simulink model "ExperimentalCarrier_lateral"  (R2015b)
settings: Solver=ode45  StartTime=0.0  StopTime=60  FixedStep=0.001  RelTol=1e-4
model workspace (MAT data in the model file):
  CX = [-0.0337179757175 -0.0333639962938 -0.0333029382182 -0.0332484475689 -0.0332754358974 -0.0333222022118 -0.0336346734879]
  CX_P = [-0.00180360991901 0.00664184177361 -2.42842311075e-05 -2.06955249234e-05 0.000107673639449 -0.00557660802406 0.00168313316358]
  CX_Q = [-0.276174674886 -0.276045033417 -0.276727133168 -0.276868141641 -0.276462581291 -0.275997191298 -0.275111306167]
  CX_R = [0.00609178533876 0.0032136083659 0.00288050935178 0.00139231210283 -0.000188148946793 -0.000699030607472 -0.00363844024964]
  CX_d = reshape([-0.0225280716674 -0.0223891508479 -0.0223681780505 -0.0223432519069 -0.0222296413505 -0.0221761942058 -0.0220710295662 0.00600012359207 0.00559383606852 0.00521927991354 0.00484253129263 0.00441803454099 0.00422262712747 0.00373799149772], [1 7 2])
  CX_d_elevator = [-0.0225280716674 -0.0223891508479 -0.0223681780505 -0.0223432519069 -0.0222296413505 -0.0221761942058 -0.0220710295662]
  CX_d_rudder = [0.00600012359207 0.00559383606852 0.00521927991354 0.00484253129263 0.00441803454099 0.00422262712747 0.00373799149772]
  CY = [0.0172529817358 0.011982932276 0.00606303689375 0.00025383868563 -0.00547298868785 -0.0111687863685 -0.0165472100647]
  CY_P = [0.374118009617 0.39290598718 0.381365334981 0.374685279781 0.377426336703 0.381898667412 0.372668227194]
  CY_Q = [0.150901852738 0.143298654224 0.128022476676 0.113476069408 0.0995119426864 0.0857134029 0.0760386872967]
  CY_R = [-0.333129286686 -0.332948508644 -0.33123397315 -0.329896924353 -0.32907206565 -0.328546079974 -0.32737851652]
  CY_d = reshape([0.0196606436595 0.0184850450981 0.0169055682098 0.0153372661358 0.0138073476115 0.0123331166649 0.0110240247349 -0.141169320798 -0.140142140967 -0.139060957332 -0.137968433842 -0.136853005187 -0.135813824899 -0.134831648888], [1 7 2])
  CY_d_elevator = [0.0196606436595 0.0184850450981 0.0169055682098 0.0153372661358 0.0138073476115 0.0123331166649 0.0110240247349]
  CY_d_rudder = [-0.141169320798 -0.140142140967 -0.139060957332 -0.137968433842 -0.136853005187 -0.135813824899 -0.134831648888]
  CZ = [0.534699164694 0.533477327658 0.533357818874 0.533162719235 0.532815330236 0.53255803197 0.533058072044]
  CZ_P = [-0.00329431835884 -0.0312298742688 -0.0131618738693 0.00139526572222 0.0131110439838 0.0227220539184 0.00563920214525]
  CZ_Q = [7.41132042869 7.41242879879 7.42202221037 7.42972491576 7.43439811242 7.43851081289 7.44797822831]
  CZ_R = [-0.0560788369874 -0.0469826195755 -0.040186761785 -0.0328451122892 -0.0248853142685 -0.0162626721689 -0.00562389662543]
  CZ_d = reshape([0.556183511159 0.556588453756 0.557396308141 0.558052886154 0.558502738673 0.558892777679 0.559544685718 -0.108954693177 -0.107634840368 -0.106474972402 -0.105298511014 -0.104084914231 -0.102894555312 -0.101853973024], [1 7 2])
  CZ_d_elevator = [0.556183511159 0.556588453756 0.557396308141 0.558052886154 0.558502738673 0.558892777679 0.559544685718]
  CZ_d_rudder = [-0.108954693177 -0.107634840368 -0.106474972402 -0.105298511014 -0.104084914231 -0.102894555312 -0.101853973024]
  Cl = [-0.00700764664959 -0.00472973282884 -0.00237582843662 -2.25913583358e-05 0.00233475877084 0.00469949778092 0.00703390515758]
  Cl_P = [-0.44204167247 -0.444124298051 -0.443158723294 -0.442636624151 -0.44302101642 -0.443480587262 -0.44220785431]
  Cl_Q = [-0.00761433176316 -0.00871202586947 -0.00915701177502 -0.00960939426583 -0.0100395709176 -0.0104261696426 -0.0111166239143]
  Cl_R = [0.0702655648896 0.0705743616107 0.0707504085215 0.0709698715526 0.0712606870971 0.0715881820975 0.0718747336385]
  Cl_d = reshape([-0.00146489638275 -0.00143738931585 -0.00137422415916 -0.00130841024919 -0.00123816152715 -0.00116289316043 -0.00109913093002 0.0123681436285 0.0122704324373 0.0121659224143 0.0120592912182 0.0119488136709 0.011839351441 0.0117379077047], [1 7 2])
  Cl_d_elevator = [-0.00146489638275 -0.00143738931585 -0.00137422415916 -0.00130841024919 -0.00123816152715 -0.00116289316043 -0.00109913093002]
  Cl_d_rudder = [0.0123681436285 0.0122704324373 0.0121659224143 0.0120592912182 0.0119488136709 0.011839351441 0.0117379077047]
  Cm = [-0.00401015961928 -0.000975274975777 -0.00046553481727 4.4136183697e-05 0.000715039140208 0.0010246745677 -0.000455960949925]
  Cm_P = [0.0363979880935 0.0870326194808 0.0380519486412 -0.00305191920923 -0.0379708477237 -0.0686773821057 -0.0415582211907]
  Cm_Q = [-9.31033666478 -9.31035016738 -9.32990293705 -9.34666189261 -9.35805453149 -9.36965047911 -9.39387328022]
  Cm_R = [0.121087302826 0.101546010828 0.0872107966775 0.0715178778578 0.0544215297596 0.0359658689904 0.0128153299816]
  Cm_d = reshape([-1.26563318748 -1.26652764985 -1.26830421062 -1.26977092408 -1.27078647089 -1.27170767282 -1.27318033181 0.238605889367 0.235644018015 0.23304116627 0.230407854048 0.227691183297 0.225077263964 0.222740695151], [1 7 2])
  Cm_d_elevator = [-1.26563318748 -1.26652764985 -1.26830421062 -1.26977092408 -1.27078647089 -1.27170767282 -1.27318033181]
  Cm_d_rudder = [0.238605889367 0.235644018015 0.23304116627 0.230407854048 0.227691183297 0.225077263964 0.222740695151]
  Cn = [0.00334100631412 0.00240143469011 0.00123926351105 0.000107729711747 -0.000988454643432 -0.00205913402605 -0.00303968727266]
  Cn_P = [-0.00770316035359 -0.00146703051444 -0.00502111646166 -0.00766050784277 -0.00674014018918 -0.00597496765186 -0.00838382166573]
  Cn_Q = [0.0596503718601 0.0577019150227 0.0528770013595 0.0482559644739 0.0438602730584 0.0395011779308 0.0366194045402]
  Cn_R = [-0.115202541198 -0.114925014185 -0.114354791039 -0.113787196313 -0.113397645546 -0.112981789027 -0.112619149701]
  Cn_d = reshape([0.00791652254186 0.00755393552521 0.00703679063877 0.00652453082009 0.00602668569172 0.00554077748029 0.00511800575953 -0.0599631923684 -0.0595911197493 -0.0591978291139 -0.0588022387871 -0.0584016103277 -0.0580069864684 -0.0576675613767], [1 7 2])
  Cn_d_elevator = [0.00791652254186 0.00755393552521 0.00703679063877 0.00652453082009 0.00602668569172 0.00554077748029 0.00511800575953]
  Cn_d_rudder = [-0.0599631923684 -0.0595911197493 -0.0591978291139 -0.0588022387871 -0.0584016103277 -0.0580069864684 -0.0576675613767]
  InertiaTensor = [1  0  0; 0  1  0; 0  0  1]
  aircraft_geometry_name = 'ExperimentalCarrier'
  alpha = 0.0912564214814
  beta = [-0.0349065850399; -0.0232710566933; -0.0116355283466; 0; 0.0116355283466; 0.0232710566933; 0.0349065850399]
  centerOfGravity = -0.092
  estimatedVelocity = 14
  mass = 1.56
  mean_chord = 0.25
  p_ini = 0
  phi_ini = 0
  psi_ini = 0
  r_ini = 0
  spanwidth = 1.5
  theta_ini = 0.0624021030233
  u_ini = 11.5418432655
  v_ini = 0
  w_ini = 1.05620086286
undefined symbols (not defined in the file): Earth, eul_0, m, pm_0, s, Vm_0, WGS84
libraries: aerolibconvert2 x6, aerolib6dofsys x2, aerolibtransform2 x2, aerolibasang x2, aerolibfltsims x2, aerolibutil x1, aerolibadyn x1, aerolibanimutils x1, aerolibatmos2 x1, aerolibgravity2 x1
settings Model: Creator=jruesch  LastModifiedBy=jruesch
settings DataIOCC: SaveFormat=Array
settings OptimizationCC: BlockReduction=off
settings HardwareCC: ProdBitPerPointer=32  ProdLargestAtomicFloat=None  ProdIntDivRoundTo=Undefined  ProdEndianess=Unspecified  ProdWordSize=32  ProdHWDeviceType=32-bit Generic
settings GRTTargetCC: GeneratePreprocessorConditionals=Disable all
settings ConfigComp: CovModelRefEnable=Off

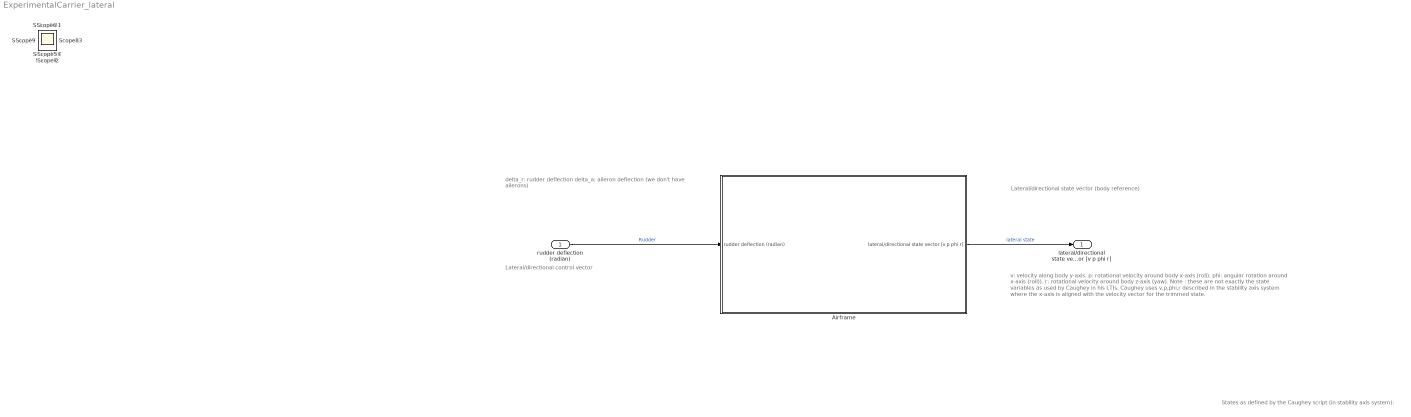
== system ExperimentalCarrier_lateral ==
  note: delta_r: rudder deflection
      | delta_a: aileron deflection (we don't have ailerons)
  note: Lateral/directional control vector
  note: v: velocity along body y-axis.
      | p: rotational velocity around body x-axis (roll).
      | phi: angular rotation around x-axis (roll)).
      | r: rotational velocity around body z-axis (yaw).
      |
      | Note : these are not exactly the state variables as used by Caughey in his LTIs.
      | Caughey uses v,p,phi,r described in the stability axis system where the x-axis is aligned
      | with the velocity vector for the trimmed state.
  note: Lateral/directional state vector (body reference)
  note: States as defined by the Caughey script (in stability axis system):
  rudder deflection (radian) : Inport
  Airframe : Subsystem
      mask Display: image(imread('../../figures/Airframe01.png'))
  lateral/directional state vector [v p phi r] : Outport
  Scope{,1..44} (45 alike) : Scope
  wires:
  rudder deflection (radian)/1 -> Airframe/1(rudder deflection (radian))  "Rudder"
  Airframe/1(lateral/directional state vector [v p phi r]) -> lateral/directional state vector [v p phi r]/1  "lateral state"

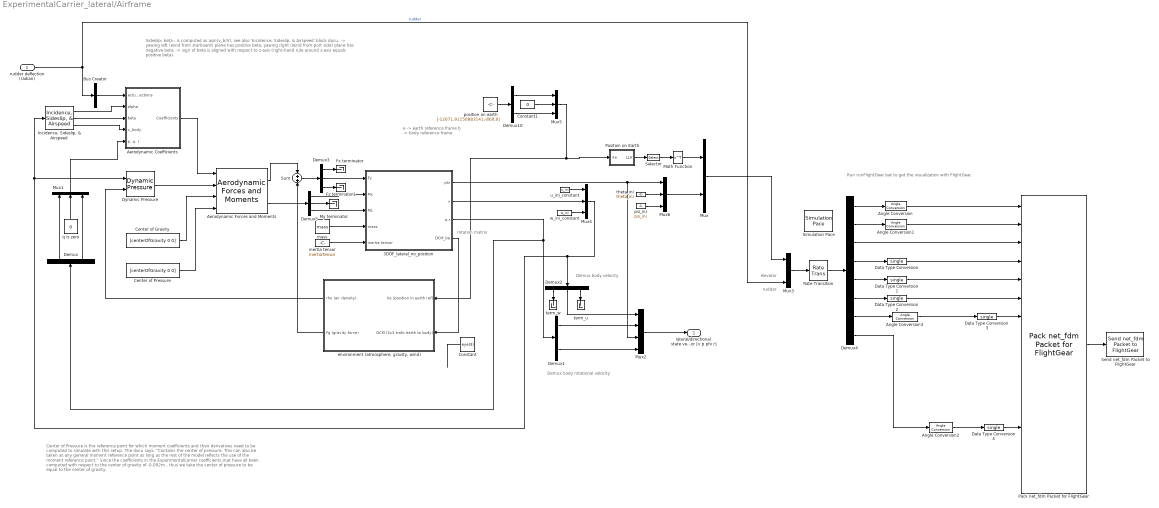
== system ExperimentalCarrier_lateral/Airframe ==
  note: rotation matrix
  note: rudder
  note: elevator
  note: Sideslip:
      | beta : is computed as asin(v_b/V), see also 'Incidence, Sideslip, & Airspeed' block docu.
      | -> yawing left (wind from starboard) plane has positive beta, yawing right (wind from port side) plane has negative beta.
      | -> sign of beta is aligned with respect to z-axis (right-hand rule around z-axis equals positive beta).
  note: Demux body velocity
  note: Run runFlightGear.bat to get the visualization with FlightGear.
  note: e -> earth reference frame
      | b -> body reference frame
  note: Center of Pressure is the reference point for which moment coefficients and their derivatives need to be computed to simulate with this setup.
      | The docu says: "Contains the center of pressure. This can also be taken as any general moment reference point as long as the rest of the model
      | reflects the use of the moment reference point." Since the coefficients in the ExperimentalCarrier coefficients.mat have all been computed with respect to
      | the center of gravity of -0.092m , thus we take the center of pressure to be equal to the center of gravity.
  note: Demux body rotational velocity
  rudder deflection (radian) : Inport
  3DOF_lateral_no_position : Subsystem
  "Aerodynamic Forces and Moments " : aerolibadyn/Aerodynamic Forces and Moments   inputAxes=Body  outputForceAxes=Body  outputMomentAxes=Body  S=spanwidth*mean_chord  b=spanwidth  cbar=mean_chord
  Aerodynamic Coefficients : Subsystem
  Angle Conversion : aerolibconvert2/Angle Conversion  IU=deg  OU=rad
  Angle Conversion1 : aerolibconvert2/Angle Conversion  IU=deg  OU=rad
  Angle Conversion2 : aerolibconvert2/Angle Conversion  IU=rad  OU=deg
  Angle Conversion3 : aerolibconvert2/Angle Conversion  IU=rad  OU=deg
  Bus Creator : BusCreator  Inputs=1
  Center of Gravity : Constant  Value=[centerOfGravity 0 0]
  Center of Pressure : Constant  Value=[centerOfGravity 0 0]
  Constant : Constant  Value=eye(3)
  Constant1 : Constant  Value=0
  Data Type Conversion{,1..4} (5 alike) : DataTypeConversion  OutDataTypeStr=single
  Demux : Demux  Outputs=2
  Demux1 : Demux  Outputs=2
  Demux10 : Demux  Outputs=2
  Demux2 : Demux  Outputs=3
  Demux3 : Demux  Outputs=3
  Demux4 : Demux  Outputs=8
  Demux5 : Demux  Outputs=3
  Dynamic Pressure : aerolibasang/Dynamic Pressure
  Fx terminator : Terminator
  Fz terminator1 : Terminator
  "Incidence, Sideslip, & Airspeed" : aerolibasang/Incidence, Sideslip, & Airspeed
  Math Function : Math  Operator=transpose  SaturateOnIntegerOverflow=on
  Mux : Mux  Inputs=2
  Mux{1,3..6} (5 alike) : Mux  Inputs=3
  Mux2 : Mux
  My terminator : Terminator
  Pack net_fdm Packet for FlightGear : aerolibfltsims/Pack net_fdm Packet for FlightGear  FlightGearVersion=v3.4  ShowPositionAttitudeInputs=on  ShowVelocityAccelerationInputs=off  ShowControlSurfacePositionInputs=on  ShowEngineFuelInputs=off  ShowLandingGearInputs=off  ShowEnvironmentInputs=off  SampleTime=1/30
  Position on Earth : Subsystem  Priority=1  TreatAsAtomicUnit=on
  Rate Transition : RateTransition  Integrity=off  OutPortSampleTime=1/30
  Selector : Selector  InputPortWidth=3  IndexOptions=Index vector (dialog)  Indices=[2 1 3]  OutputSizes=1
  Send net_fdm Packet to FlightGear : aerolibfltsims/Send net_fdm Packet to FlightGear  DestinationIpAddress=127.0.0.1  DestinationPort=5502  LocalIpPort=-1  varLen=off  SampleTime=1/30
  Simulation Pace : aerolibanimutils/Simulation Pace  SimulationPace=1  SleepMode=MATLAB Thread  OutputPaceError=off  SampleTime=1/30
      settings: AttributesFormatString=%<SimulationPace> sec/sec
  Sum : Sum
  "environment (atmosphere, gravity, wind)" : Subsystem
  inertia tensor : Constant  Value=InertiaTensor
  mass : Constant  Value=mass
  position on earth : Constant  Value=[-12071.91150883141;-800.0]
  psi_ini : Constant  Value=psi_ini
  q is zero : Constant  Value=0
  term_u : Terminator
  term_w : Terminator
  theta_ini : Constant  Value=theta_ini
  u_ini_constant : Constant  Value=u_ini
  w_ini_constant : Constant  Value=w_ini
  lateral/directional state vector [v p phi r] : Outport
  wires:
  "Aerodynamic Forces and Moments "/1 -> Sum/1
  "Aerodynamic Forces and Moments "/2 -> Demux5/1
  Center of Gravity/1 -> "Aerodynamic Forces and Moments "/3
  Center of Pressure/1 -> "Aerodynamic Forces and Moments "/4
  Dynamic Pressure/1 -> "Aerodynamic Forces and Moments "/2
  Position on Earth/1(LLA) -> Selector/1
  3DOF_lateral_no_position/4(DCM_be) -> "environment (atmosphere, gravity, wind)"/2(DCM (3x3 trafo earth to body))
  3DOF_lateral_no_position/1(phi) -> Mux6/1, Mux2/3
  Mux4/1 -> Demux2/1, "Incidence, Sideslip, & Airspeed"/1, Dynamic Pressure/1
  3DOF_lateral_no_position/3(p,r) -> Demux/1, Demux1/1
  Math Function/1 -> Mux/1
  Mux/1 -> Mux3/1
  Selector/1 -> Math Function/1
  "environment (atmosphere, gravity, wind)"/1(rho (air density)) -> Dynamic Pressure/2
  "environment (atmosphere, gravity, wind)"/2(Fg (gravity force)) -> Sum/2
  "Incidence, Sideslip, & Airspeed"/2 -> Aerodynamic Coefficients/3(beta)
  "Incidence, Sideslip, & Airspeed"/3 -> Aerodynamic Coefficients/4(v_body)
  Aerodynamic Coefficients/1(Coefficients) -> "Aerodynamic Forces and Moments "/1
  Bus Creator/1 -> Aerodynamic Coefficients/1(actuator deflections)
  rudder deflection (radian)/1 -> Bus Creator/1, Mux3/3  "rudder"
  Sum/1 -> Demux3/1
  Demux1/1 -> Mux2/2
  Mux2/1 -> lateral/directional state vector [v p phi r]/1
  Pack net_fdm Packet for FlightGear/1 -> Send net_fdm Packet to FlightGear/1
  Demux4/1 -> Angle Conversion/1
  Demux4/2 -> Angle Conversion1/1
  Demux4/3 -> Pack net_fdm Packet for FlightGear/3
  Demux4/4 -> Data Type Conversion/1
  Demux4/5 -> Data Type Conversion1/1
  Demux4/6 -> Data Type Conversion2/1
  Rate Transition/1 -> Demux4/1
  Angle Conversion/1 -> Pack net_fdm Packet for FlightGear/1
  Angle Conversion1/1 -> Pack net_fdm Packet for FlightGear/2
  Data Type Conversion/1 -> Pack net_fdm Packet for FlightGear/4
  Data Type Conversion1/1 -> Pack net_fdm Packet for FlightGear/5
  Data Type Conversion2/1 -> Pack net_fdm Packet for FlightGear/6
  Mux3/1 -> Rate Transition/1
  Demux4/7 -> Angle Conversion3/1
  Demux4/8 -> Angle Conversion2/1
  Data Type Conversion3/1 -> Pack net_fdm Packet for FlightGear/7
  Data Type Conversion4/1 -> Pack net_fdm Packet for FlightGear/13
  Angle Conversion2/1 -> Data Type Conversion4/1
  Angle Conversion3/1 -> Data Type Conversion3/1
  inertia tensor/1 -> 3DOF_lateral_no_position/5(inertia tensor)
  mass/1 -> 3DOF_lateral_no_position/4("mass ")
  Constant1/1 -> Mux5/2
  position on earth/1 -> Demux10/1
  Demux10/2 -> Mux5/3
  Demux10/1 -> Mux5/1
  Mux5/1 -> Position on Earth/1(Xe), "environment (atmosphere, gravity, wind)"/1(Xe (position in earth ref))
  Demux3/2 -> 3DOF_lateral_no_position/1(Fy)
  Demux5/1 -> 3DOF_lateral_no_position/2(Mx)
  Demux5/3 -> 3DOF_lateral_no_position/3(Mz)
  Demux5/2 -> My terminator/1
  Demux3/1 -> Fx terminator/1
  Demux3/3 -> Fz terminator1/1
  Demux1/2 -> Mux2/4
  Demux/1 -> Mux1/1
  Demux/2 -> Mux1/3
  Mux1/1 -> Aerodynamic Coefficients/5("p, q, r")
  q is zero/1 -> Mux1/2
  w_ini_constant/1 -> Mux4/3
  u_ini_constant/1 -> Mux4/1
  3DOF_lateral_no_position/2(v) -> Mux4/2
  theta_ini/1 -> Mux6/2
  psi_ini/1 -> Mux6/3
  Mux6/1 -> Mux/2
  Demux2/2 -> Mux2/1
  Demux2/1 -> term_w/1
  Demux2/3 -> term_u/1
  Constant/1 -> ?
  "Incidence, Sideslip, & Airspeed"/1 -> Aerodynamic Coefficients/2(alpha)

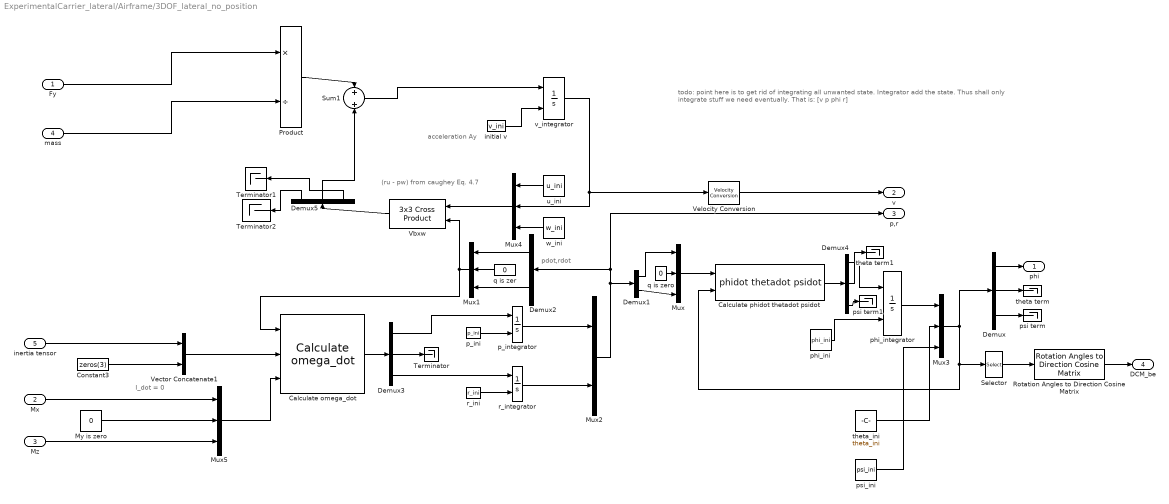
== system ExperimentalCarrier_lateral/Airframe/3DOF_lateral_no_position ==
  note: (ru - pw)
      | from caughey Eq. 4.7
  note: I_dot = 0
  note: todo: point here is to get rid of integrating all unwanted state.
      | Integrator add the state. Thus shall only integrate stuff we need
      | eventually. That is: [v p phi r]
  note: pdot,rdot
  note: acceleration Ay
  Fy : Inport
  Mx : Inport  Port=2  PortDimensions=1
  Mz : Inport  Port=3  PortDimensions=1
  "mass " : Inport  Port=4
  inertia tensor : Inport  Port=5
  Calculate omega_dot : aerolib6dofsys/Calculate omega_dot  SystemSampleTime=-1
  Calculate phidot thetadot psidot : aerolib6dofsys/DCM & Euler Angles (Euler)/phidot thetadot psidot
  Constant3 : Constant  Value=zeros(3)
  Demux{,3..5} (4 alike) : Demux  Outputs=3
  Demux1 : Demux  Outputs=2
  Demux2 : Demux  Outputs=2
  Mux{,1,3..5} (5 alike) : Mux  Inputs=3
  Mux2 : Mux  Inputs=2
  My is zero : Constant  Value=0
  Product : Product  Inputs=*/  SaturateOnIntegerOverflow=on  OutDataTypeStr=Inherit: Same as first input
  Rotation Angles to Direction Cosine Matrix : aerolibtransform2/Rotation Angles to Direction Cosine Matrix  rotationOrder=ZYX
  Selector : Selector  InputPortWidth=3  IndexOptions=Index vector (dialog)  Indices=[3 2 1]  OutputSizes=1
  Sum1 : Sum  SaturateOnIntegerOverflow=on
  Terminator : Terminator
  Terminator1 : Terminator
  Terminator2 : Terminator
  Vbxw : aerolibutil/3x3 Cross Product
  Vector Concatenate1 : Concatenate  Mode=Multidimensional array
  Velocity Conversion : aerolibconvert2/Velocity Conversion  IU=m/s  OU=m/s
  initial v : Constant  Value=v_ini
  p_ini : Constant  Value=p_ini
  p_integrator : Integrator  InitialConditionSource=external  InitialCondition=pm_0
  phi_ini : Constant  Value=phi_ini
  phi_integrator : Integrator  InitialConditionSource=external  InitialCondition=eul_0
  psi term : Terminator
  psi term1 : Terminator
  psi_ini : Constant  Value=psi_ini
  q is zer : Constant  Value=0
  q is zero : Constant  Value=0
  r_ini : Constant  Value=r_ini
  r_integrator : Integrator  InitialConditionSource=external  InitialCondition=pm_0
  theta term : Terminator
  theta term1 : Terminator
  theta_ini : Constant  Value=theta_ini
  u_ini : Constant  Value=u_ini
  v_integrator : Integrator  InitialConditionSource=external  InitialCondition=Vm_0
  w_ini : Constant  Value=w_ini
  phi : Outport
  v : Outport  Port=2
  p,r : Outport  Port=3
  DCM_be : Outport  Port=4
  wires:
  Sum1/1 -> v_integrator/1
  v_integrator/1 -> Mux4/2, Velocity Conversion/1
  Velocity Conversion/1 -> v/1
  Calculate phidot thetadot psidot/1 -> Demux4/1
  Product/1 -> Sum1/1
  Fy/1 -> Product/1
  Mx/1 -> Mux5/1
  p_integrator/1 -> Mux2/1
  Vbxw/1 -> Demux5/1
  inertia tensor/1 -> Vector Concatenate1/1
  "mass "/1 -> Product/2
  Mux5/1 -> Calculate omega_dot/3
  p_ini/1 -> p_integrator/2
  initial v/1 -> v_integrator/2
  Rotation Angles to Direction Cosine Matrix/1 -> DCM_be/1
  Selector/1 -> Rotation Angles to Direction Cosine Matrix/1
  Mz/1 -> Mux5/3
  Demux/1 -> phi/1
  Demux/2 -> theta term/1
  Demux/3 -> psi term/1
  Mux/1 -> Calculate phidot thetadot psidot/1
  Demux1/1 -> Mux/1
  Demux1/2 -> Mux/3
  q is zero/1 -> Mux/2
  Vector Concatenate1/1 -> Calculate omega_dot/2
  Constant3/1 -> Vector Concatenate1/2
  My is zero/1 -> Mux5/2
  q is zer/1 -> Mux1/2
  Demux2/1 -> Mux1/1
  Demux2/2 -> Mux1/3
  Mux1/1 -> Vbxw/2, Calculate omega_dot/1
  Calculate omega_dot/1 -> Demux3/1
  Demux3/2 -> Terminator/1
  Demux3/1 -> p_integrator/1
  Demux3/3 -> r_integrator/1
  Demux4/1 -> phi_integrator/1
  Mux3/1 -> Demux/1, Calculate phidot thetadot psidot/2, Selector/1
  phi_integrator/1 -> Mux3/1
  Demux4/2 -> theta term1/1
  Demux4/3 -> psi term1/1
  phi_ini/1 -> phi_integrator/2
  psi_ini/1 -> Mux3/3
  theta_ini/1 -> Mux3/2
  Mux4/1 -> Vbxw/1
  u_ini/1 -> Mux4/1
  w_ini/1 -> Mux4/3
  Demux5/2 -> Sum1/2
  Demux5/3 -> Terminator1/1
  Demux5/1 -> Terminator2/1
  r_ini/1 -> r_integrator/2
  Mux2/1 -> Demux2/1, p,r/1, Demux1/1
  r_integrator/1 -> Mux2/2

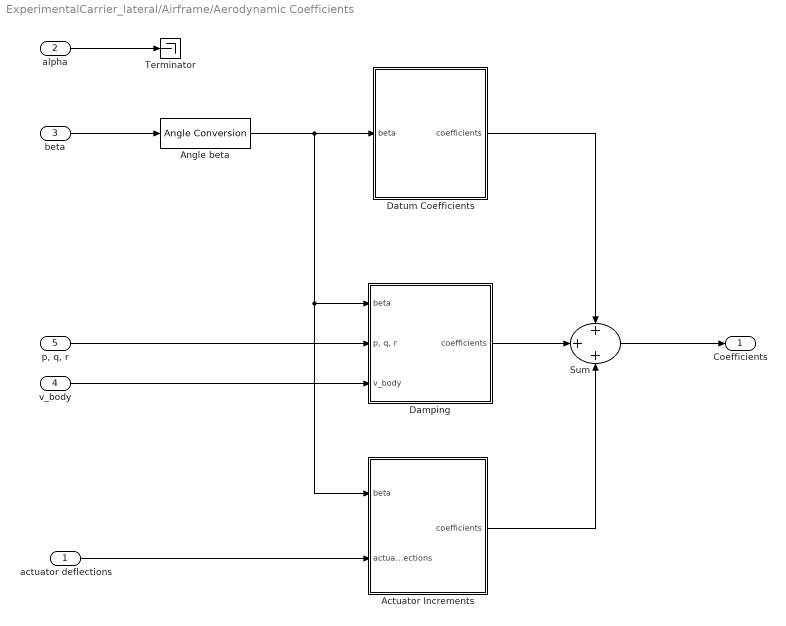
== system ExperimentalCarrier_lateral/Airframe/Aerodynamic Coefficients ==
  actuator deflections : Inport
  alpha : Inport  Port=2
  beta : Inport  Port=3
  v_body : Inport  Port=4
  "p, q, r" : Inport  Port=5
  Actuator Increments : Subsystem
  Angle beta : aerolibconvert2/Angle Conversion  IU=rad  OU=deg
  Damping : Subsystem
  Datum Coefficients : Subsystem
  Sum : Sum  Inputs=+++
  Terminator : Terminator
  Coefficients : Outport
  wires:
  Angle beta/1 -> Actuator Increments/1(beta), Damping/1(beta), Datum Coefficients/1(beta)
  Datum Coefficients/1(coefficients) -> Sum/1
  "p, q, r"/1 -> Damping/2("p, q, r")
  Damping/1(coefficients) -> Sum/2
  Sum/1 -> Coefficients/1
  v_body/1 -> Damping/3(v_body)
  beta/1 -> Angle beta/1
  actuator deflections/1 -> Actuator Increments/2(actuator deflections)
  Actuator Increments/1(coefficients) -> Sum/3
  alpha/1 -> Terminator/1

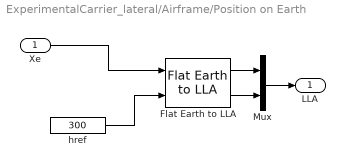
== system ExperimentalCarrier_lateral/Airframe/Position on Earth ==
  Xe : Inport
  Flat Earth to LLA : aerolibtransform2/Flat Earth to LLA  units=Metric (MKS)  ptype=Earth (WGS84)  F=1/298.257223563  R=6378137  LL0=[37.628738616666666,-1.223933911333333e+02]  psi=0
  Mux : Mux  Inputs=2
  href : Constant  Value=300
  LLA : Outport
  wires:
  Mux/1 -> LLA/1
  Xe/1 -> Flat Earth to LLA/1
  Flat Earth to LLA/1 -> Mux/1
  Flat Earth to LLA/2 -> Mux/2
  href/1 -> Flat Earth to LLA/2

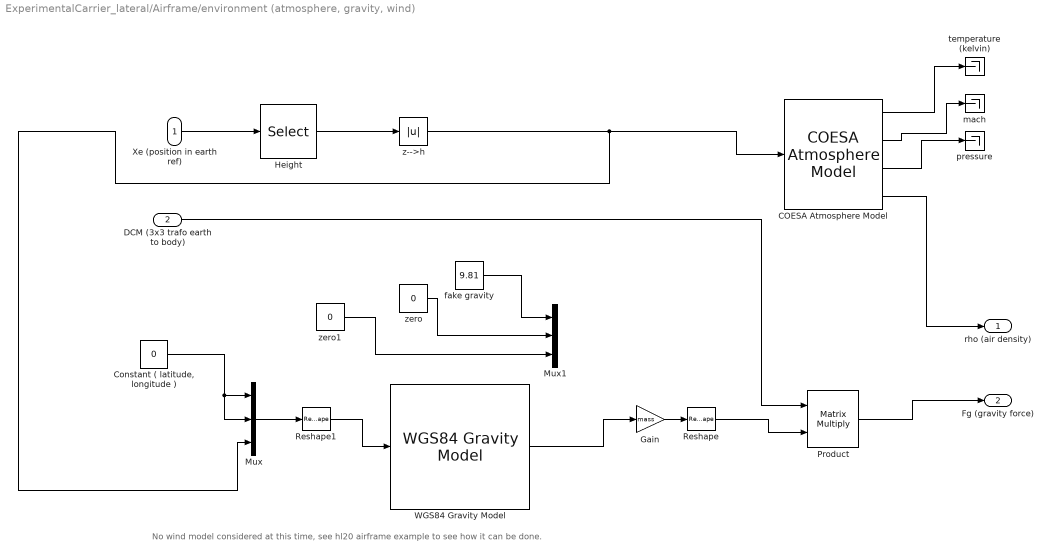
== system ExperimentalCarrier_lateral/Airframe/environment (atmosphere, gravity, wind) ==
  note: No wind model considered at this time, see hl20 airframe example to see how it can be done.
  Xe (position in earth ref) : Inport
  DCM (3x3 trafo earth to body) : Inport  Port=2
  COESA Atmosphere Model : aerolibatmos2/COESA Atmosphere Model  units=Metric (MKS)  spec=1976 COESA-extended U.S. Standard Atmosphere  model=Profile  profile_var=High temperature  profile_percent=1%  profile_alt=5 km (16404 ft)  envelope_var=High temperature  envelope_percent=1%  action=Warning
  "Constant ( latitude, longitude )" : Constant  Value=0
  Gain : Gain  Gain=mass
  Height : Selector  InputPortWidth=3  IndexOptions=Index vector (dialog)  Indices=[3]  OutputSizes=1
  Mux : Mux  Inputs=3
  Mux1 : Mux  Inputs=3
  Product : Product  Multiplication=Matrix(*)
  Reshape : Reshape
  Reshape1 : Reshape
  "WGS84 Gravity Model " : aerolibgravity2/WGS84 Gravity Model   model=WGS84 Taylor Series  units=Metric (MKS)  no_atmos=on  precessing=on  jd_loc=off  month=October  day=10  year=2004  no_centrifugal=on  action=Warning
  fake gravity : Constant  Value=9.81
  mach : Terminator
  pressure : Terminator
  temperature (kelvin) : Terminator
  z-->h : Abs  SaturateOnIntegerOverflow=on
  zero : Constant  Value=0
  zero1 : Constant  Value=0
  rho (air density) : Outport
  Fg (gravity force) : Outport  Port=2
  wires:
  Xe (position in earth ref)/1 -> Height/1
  Height/1 -> z-->h/1
  z-->h/1 -> Mux/3, COESA Atmosphere Model/1
  COESA Atmosphere Model/4 -> rho (air density)/1
  COESA Atmosphere Model/1 -> temperature (kelvin)/1
  COESA Atmosphere Model/2 -> mach/1
  COESA Atmosphere Model/3 -> pressure/1
  "Constant ( latitude, longitude )"/1 -> Mux/1, Mux/2
  Mux/1 -> Reshape1/1
  fake gravity/1 -> Mux1/1
  Gain/1 -> Reshape/1
  Reshape/1 -> Product/2
  DCM (3x3 trafo earth to body)/1 -> Product/1
  Product/1 -> Fg (gravity force)/1
  zero/1 -> Mux1/2
  zero1/1 -> Mux1/3
  Reshape1/1 -> "WGS84 Gravity Model "/1
  "WGS84 Gravity Model "/1 -> Gain/1

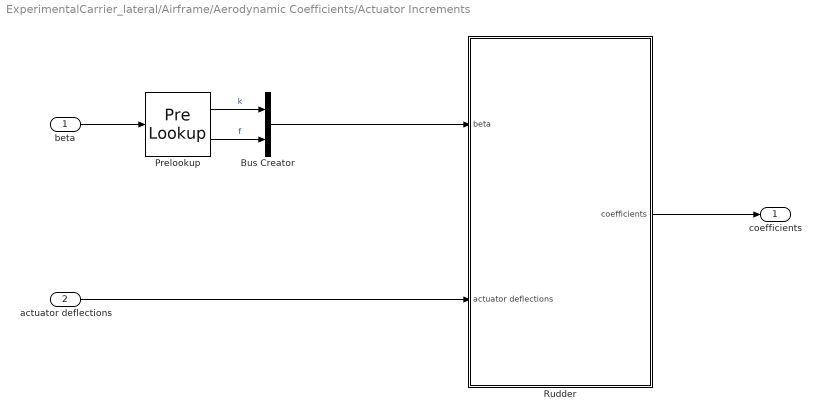
== system ExperimentalCarrier_lateral/Airframe/Aerodynamic Coefficients/Actuator Increments ==
  beta : Inport
  actuator deflections : Inport  Port=2
  Bus Creator : BusCreator  Inputs=2
  Prelookup : PreLookup  BreakpointsData=beta*180/pi  ExtrapMethod=Linear
  Rudder : Subsystem
  coefficients : Outport
  wires:
  beta/1 -> Prelookup/1
  actuator deflections/1 -> Rudder/2(actuator deflections)
  Bus Creator/1 -> Rudder/1(beta)
  Prelookup/1 -> Bus Creator/1  "k"
  Prelookup/2 -> Bus Creator/2  "f"
  Rudder/1(coefficients) -> coefficients/1

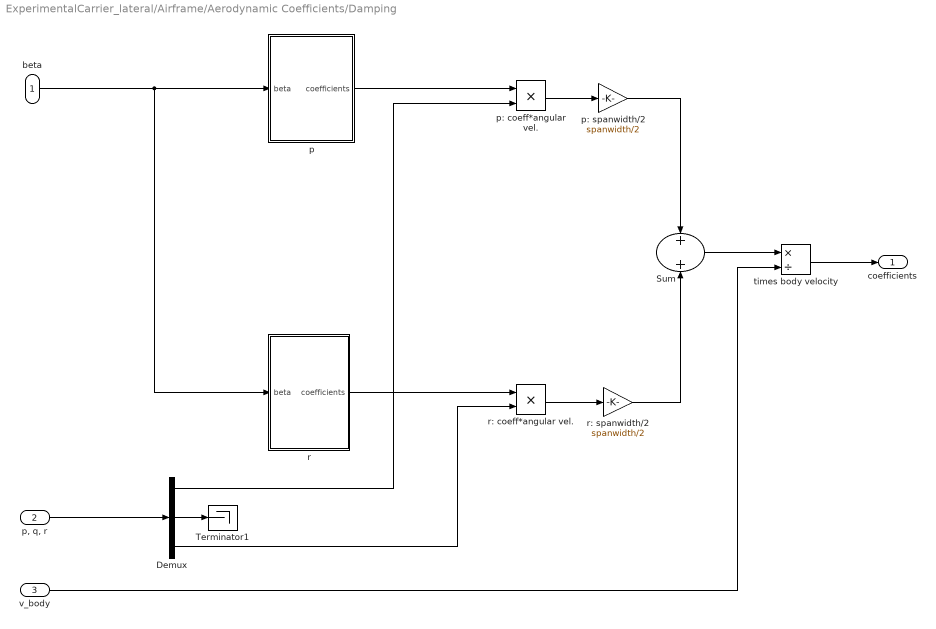
== system ExperimentalCarrier_lateral/Airframe/Aerodynamic Coefficients/Damping ==
  beta : Inport
  "p, q, r" : Inport  Port=2
  v_body : Inport  Port=3
  Demux : Demux  Outputs=3
  Sum : Sum
  Terminator1 : Terminator
  p : Subsystem
  p: coeff*angular vel. : Product
  p: spanwidth/2 : Gain  Gain=spanwidth/2
  r : Subsystem
  r: coeff*angular vel. : Product
  r: spanwidth/2 : Gain  Gain=spanwidth/2
  times body velocity : Product  Inputs=*/
  coefficients : Outport
  wires:
  beta/1 -> r/1(beta), p/1(beta)
  p/1(coefficients) -> p: coeff*angular vel./1
  "p, q, r"/1 -> Demux/1
  p: coeff*angular vel./1 -> p: spanwidth/2/1
  p: spanwidth/2/1 -> Sum/1
  Sum/1 -> times body velocity/1
  v_body/1 -> times body velocity/2
  r/1(coefficients) -> r: coeff*angular vel./1
  r: spanwidth/2/1 -> Sum/2
  r: coeff*angular vel./1 -> r: spanwidth/2/1
  times body velocity/1 -> coefficients/1
  Demux/1 -> p: coeff*angular vel./2
  Demux/3 -> r: coeff*angular vel./2
  Demux/2 -> Terminator1/1

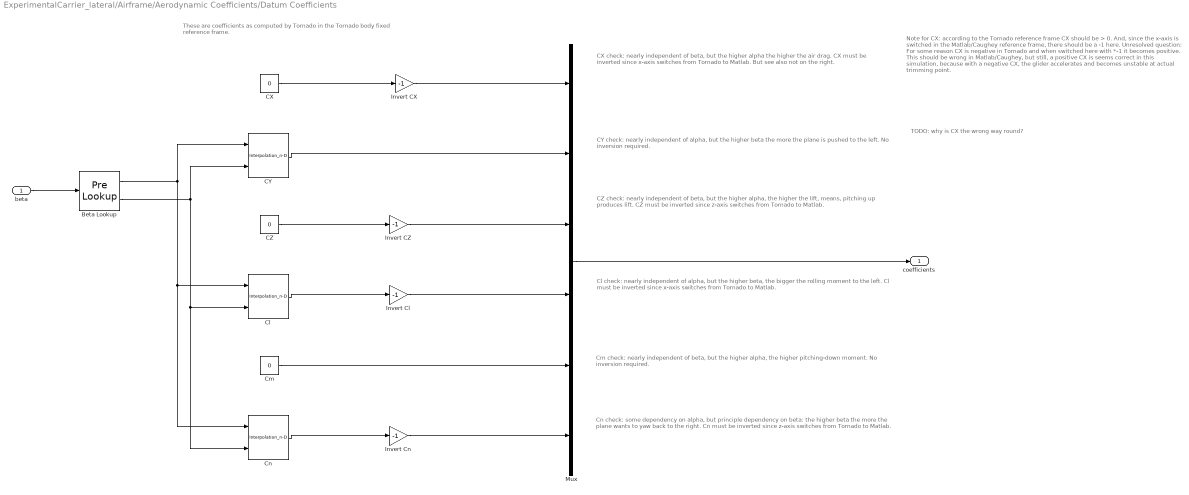
== system ExperimentalCarrier_lateral/Airframe/Aerodynamic Coefficients/Datum Coefficients ==
  note: Cl check: nearly independent of alpha, but the higher beta, the bigger the rolling moment to the left. Cl must be inverted since x-axis switches from Tornado to Matlab.
  note: CY check: nearly independent of alpha, but
      | the higher beta the more the plane is pushed to the left. No inversion required.
  note: These are coefficients as computed by Tornado in the
      | Tornado body fixed reference frame.
  note: Cm check: nearly independent of beta, but the higher alpha, the higher pitching-down moment. No inversion required.
  note: CZ check: nearly independent of beta, but the higher alpha, the higher the lift, means, pitching up produces lift. CZ must be inverted since z-axis switches from Tornado to Matlab.
  note: Note for CX: according to the Tornado reference frame
      | CX should be > 0. And, since the x-axis is switched in the
      | Matlab/Caughey reference frame, there should be a -1 here.
      | Unresolved question: For some reason CX is negative in Tornado
      | and when switched here with *-1 it becomes positive. This should
      | be wrong in Matlab/Caughey, but still, a positive CX is seems correct
      | in this simulation, because with a negative CX, the glider
      | accelerates and becomes unstable at actual trimming point.
  note: Cn check: some dependency on alpha, but principle dependency on beta: the higher beta the more the plane wants to yaw back to the right. Cn must be inverted since z-axis switches from Tornado to Matlab.
  note: CX check: nearly independent of beta, but the higher alpha the higher the air drag. CX must be inverted since x-axis switches from Tornado to Matlab. But see also not on the right.
  note: TODO:
      | why is CX the wrong way round?
  beta : Inport
  Beta Lookup : PreLookup  BreakpointsData=beta*180/pi  ExtrapMethod=Linear
  CX : Constant  Value=0
  CY : Interpolation_n-D  NumberOfTableDimensions=1  Table=CY  InternalRulePriority=Speed
      settings: InputPortMap=u0,u1
  CZ : Constant  Value=0
  Cl : Interpolation_n-D  NumberOfTableDimensions=1  Table=Cl  InternalRulePriority=Speed
      settings: InputPortMap=u0,u1
  Cm : Constant  Value=0
  Cn : Interpolation_n-D  NumberOfTableDimensions=1  Table=Cn  InternalRulePriority=Speed
      settings: InputPortMap=u0,u1
  Invert CX : Gain  Gain=-1
  Invert CZ : Gain  Gain=-1
  Invert Cl : Gain  Gain=-1
  Invert Cn : Gain  Gain=-1
  Mux : Mux  Inputs=6
  coefficients : Outport
  wires:
  Beta Lookup/1 -> CY/1, Cn/1, Cl/1
  Beta Lookup/2 -> Cn/2, Cl/2, CY/2
  beta/1 -> Beta Lookup/1
  Mux/1 -> coefficients/1
  CZ/1 -> Invert CZ/1
  CY/1 -> Mux/2
  CX/1 -> Invert CX/1
  Cl/1 -> Invert Cl/1
  Cn/1 -> Invert Cn/1
  Invert CZ/1 -> Mux/3
  Invert Cl/1 -> Mux/4
  Invert Cn/1 -> Mux/6
  Invert CX/1 -> Mux/1
  Cm/1 -> Mux/5

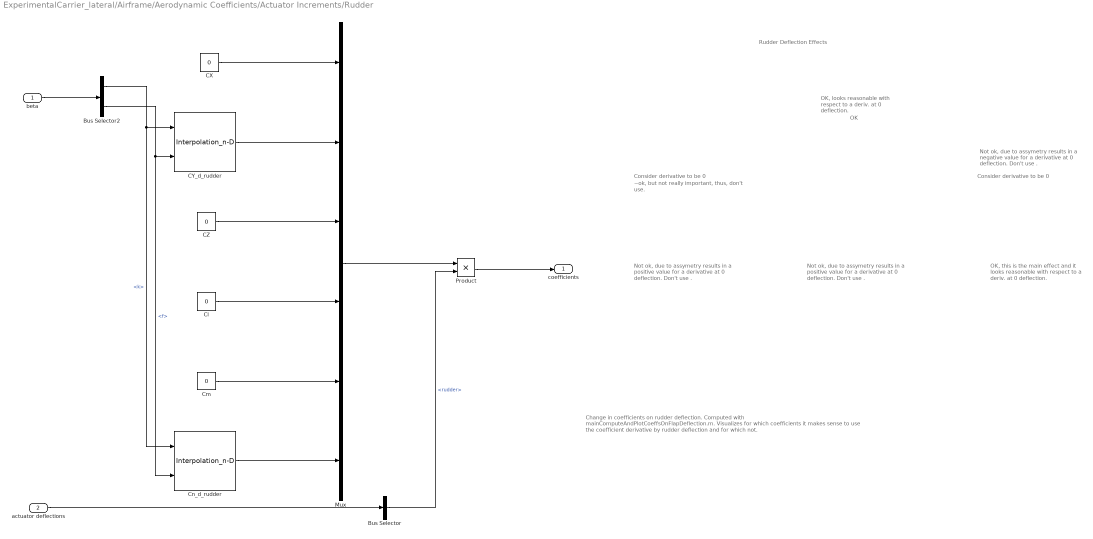
== system ExperimentalCarrier_lateral/Airframe/Aerodynamic Coefficients/Actuator Increments/Rudder ==
  note: Consider derivative to be 0
  note: Consider derivative to be 0
  note: OK
  note: Not ok, due to assymetry
      | results in a positive
      | value for a derivative at 0
      | deflection. Don't use .
  note: Not ok, due to assymetry
      | results in a positive
      | value for a derivative at 0
      | deflection. Don't use .
  note: OK, this is the main effect
      | and it looks reasonable
      | with respect to a deriv.
      | at 0 deflection.
  note: Not ok, due to assymetry
      | results in a negative
      | value for a derivative at 0
      | deflection. Don't use .
  note: OK, looks reasonable
      | with respect to a deriv.
      | at 0 deflection.
  note: ~ok, but not really important,
      | thus, don't use.
  note: Change in coefficients on rudder deflection. Computed with mainComputeAndPlotCoeffsOnFlapDeflection.m.
      | Visualizes for which coefficients it makes sense to use the coefficient derivative by rudder deflection and for which not.
  note: Rudder Deflection Effects
  beta : Inport
  actuator deflections : Inport  Port=2
  Bus Selector : BusSelector  OutputSignals=rudder
  Bus Selector2 : BusSelector  OutputSignals=k,f
  CX : Constant  Value=0
  CY_d_rudder : Interpolation_n-D  NumberOfTableDimensions=1  Table=CY_d_rudder  InternalRulePriority=Speed
      settings: InputPortMap=u0,u1
  CZ : Constant  Value=0
  Cl : Constant  Value=0
  Cm : Constant  Value=0
  Cn_d_rudder : Interpolation_n-D  NumberOfTableDimensions=1  Table=Cn_d_rudder  InternalRulePriority=Speed
      settings: InputPortMap=u0,u1
  Mux : Mux  Inputs=6
  Product : Product
  coefficients : Outport
  wires:
  Bus Selector2/1 -> Cn_d_rudder/1, CY_d_rudder/1  "<k>"
  Bus Selector2/2 -> Cn_d_rudder/2, CY_d_rudder/2  "<f>"
  CX/1 -> Mux/1
  CY_d_rudder/1 -> Mux/2
  CZ/1 -> Mux/3
  Cl/1 -> Mux/4
  Cn_d_rudder/1 -> Mux/6
  actuator deflections/1 -> Bus Selector/1
  Product/1 -> coefficients/1
  Bus Selector/1 -> Product/2  "<rudder>"
  Mux/1 -> Product/1
  beta/1 -> Bus Selector2/1
  Cm/1 -> Mux/5

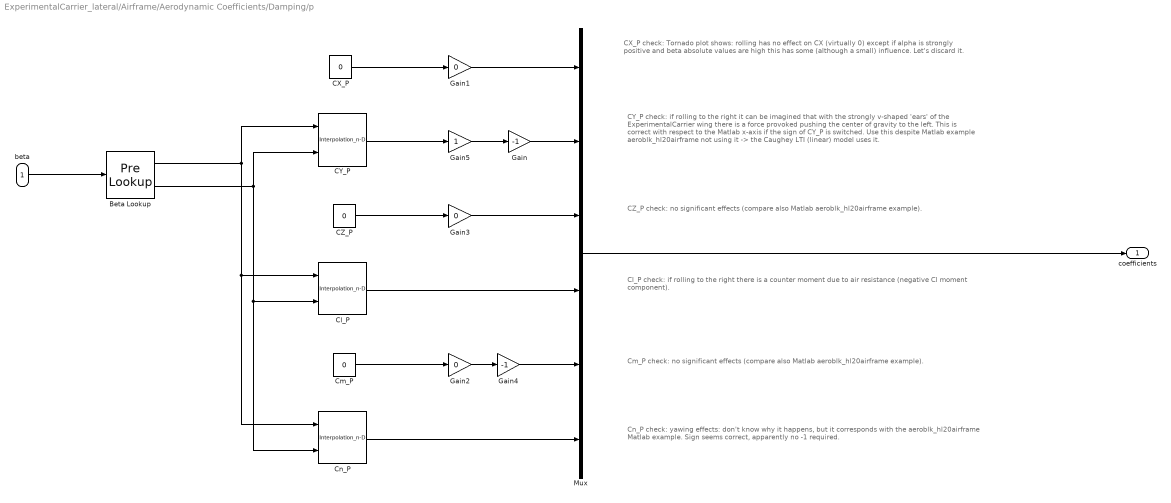
== system ExperimentalCarrier_lateral/Airframe/Aerodynamic Coefficients/Damping/p ==
  note: Cn_P check: yawing effects: don't know why it happens, but it corresponds with the aeroblk_hl20airframe Matlab example. Sign seems correct, apparently no -1 required.
  note: CZ_P check: no significant effects (compare also Matlab aeroblk_hl20airframe example).
  note: Cl_P check: if rolling to the right there is a counter moment due to air resistance (negative Cl moment component).
  note: CY_P check: if rolling to the right it can be imagined that with the strongly v-shaped 'ears' of the ExperimentalCarrier wing there is a force provoked pushing the center of gravity to the left. This is correct with respect to the Matlab x-axis if the sign of CY_P is switched. Use this despite Matlab example aeroblk_hl20airframe not using it -> the Caughey LTI (linear) model uses it.
  note: CX_P check: Tornado plot shows: rolling has no effect on CX (virtually 0) except if alpha is strongly positive and beta absolute values are high this has some (although a small) influence. Let's discard it.
  note: Cm_P check: no significant effects (compare also Matlab aeroblk_hl20airframe example).
  beta : Inport
  Beta Lookup : PreLookup  BreakpointsData=beta*180/pi  ExtrapMethod=Linear
  CX_P : Constant  Value=0
  CY_P : Interpolation_n-D  NumberOfTableDimensions=1  Table=CY_P  InternalRulePriority=Speed
      settings: InputPortMap=u0,u1
  CZ_P : Constant  Value=0
  Cl_P : Interpolation_n-D  NumberOfTableDimensions=1  Table=Cl_P  InternalRulePriority=Speed
      settings: InputPortMap=u0,u1
  Cm_P : Constant  Value=0
  Cn_P : Interpolation_n-D  NumberOfTableDimensions=1  Table=Cn_P  InternalRulePriority=Speed
      settings: InputPortMap=u0,u1
  Gain : Gain  Gain=-1
  Gain1 : Gain  Gain=0
  Gain2 : Gain  Gain=0
  Gain3 : Gain  Gain=0
  Gain4 : Gain  Gain=-1
  Gain5 : Gain
  Mux : Mux  Inputs=6
  coefficients : Outport
  wires:
  Beta Lookup/2 -> Cn_P/2, Cl_P/2, CY_P/2
  CX_P/1 -> Gain1/1
  Beta Lookup/1 -> Cn_P/1, Cl_P/1, CY_P/1
  beta/1 -> Beta Lookup/1
  CY_P/1 -> Gain5/1
  CZ_P/1 -> Gain3/1
  Cl_P/1 -> Mux/4
  Cn_P/1 -> Mux/6
  Mux/1 -> coefficients/1
  Gain/1 -> Mux/2
  Cm_P/1 -> Gain2/1
  Gain1/1 -> Mux/1
  Gain2/1 -> Gain4/1
  Gain3/1 -> Mux/3
  Gain4/1 -> Mux/5
  Gain5/1 -> Gain/1

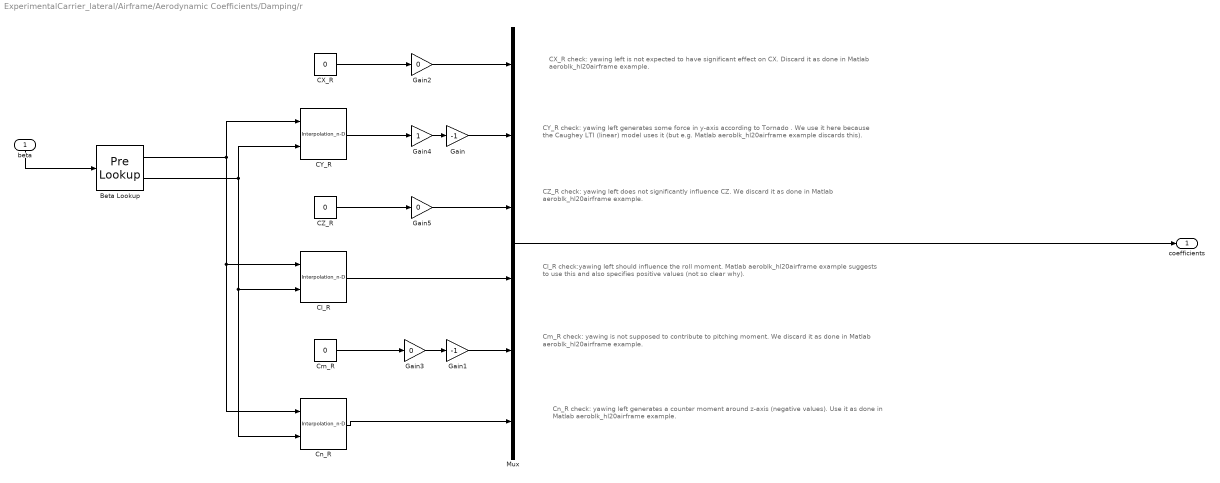
== system ExperimentalCarrier_lateral/Airframe/Aerodynamic Coefficients/Damping/r ==
  note: Cn_R check: yawing left generates a counter moment around z-axis (negative values). Use it as done in Matlab aeroblk_hl20airframe example.
  note: Cm_R check: yawing is not supposed to contribute to pitching moment. We discard it as done in Matlab aeroblk_hl20airframe example.
  note: Cl_R check:yawing left should influence the roll moment. Matlab aeroblk_hl20airframe example suggests to use this and also specifies positive values (not so clear why).
  note: CZ_R check: yawing left does not significantly influence CZ. We discard it as done in Matlab aeroblk_hl20airframe example.
  note: CY_R check: yawing left generates some force in y-axis according to Tornado . We use it here
      | because the Caughey LTI (linear) model uses it (but e.g. Matlab aeroblk_hl20airframe example discards this).
  note: CX_R check: yawing left is not expected to have significant effect on CX. Discard it as done in Matlab aeroblk_hl20airframe example.
  beta : Inport
  Beta Lookup : PreLookup  BreakpointsData=beta*180/pi  ExtrapMethod=Linear
  CX_R : Constant  Value=0
  CY_R : Interpolation_n-D  NumberOfTableDimensions=1  Table=CY_R  InternalRulePriority=Speed
      settings: InputPortMap=u0,u1
  CZ_R : Constant  Value=0
  Cl_R : Interpolation_n-D  NumberOfTableDimensions=1  Table=Cl_R  InternalRulePriority=Speed
      settings: InputPortMap=u0,u1
  Cm_R : Constant  Value=0
  Cn_R : Interpolation_n-D  NumberOfTableDimensions=1  Table=Cn_R  InternalRulePriority=Speed
      settings: InputPortMap=u0,u1
  Gain : Gain  Gain=-1
  Gain1 : Gain  Gain=-1
  Gain2 : Gain  Gain=0
  Gain3 : Gain  Gain=0
  Gain4 : Gain
  Gain5 : Gain  Gain=0
  Mux : Mux  Inputs=6
  coefficients : Outport
  wires:
  CZ_R/1 -> Gain5/1
  CY_R/1 -> Gain4/1
  Cm_R/1 -> Gain3/1
  Cl_R/1 -> Mux/4
  beta/1 -> Beta Lookup/1
  Beta Lookup/1 -> CY_R/1, Cn_R/1, Cl_R/1
  Beta Lookup/2 -> CY_R/2, Cn_R/2, Cl_R/2
  Cn_R/1 -> Mux/6
  Mux/1 -> coefficients/1
  CX_R/1 -> Gain2/1
  Gain/1 -> Mux/2
  Gain1/1 -> Mux/5
  Gain2/1 -> Mux/1
  Gain3/1 -> Gain1/1
  Gain4/1 -> Gain/1
  Gain5/1 -> Mux/3
